simulink model "W04_1_straight"  (R2024b)
settings: Solver=FixedStepDiscrete  StartTime=0.0  StopTime=inf  FixedStep=0.05  RelTol=1e-3
values from neighbouring files (symbols this model uses):
  animate = 1    [W04_setup.m]
libraries: ros2lib x5
settings Model: Creator=admin  LastModifiedBy=admin

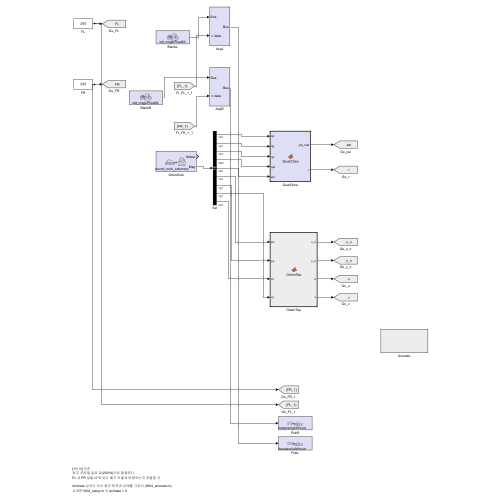
[thumbnail: Simulink's stored preview of the top-level diagram]
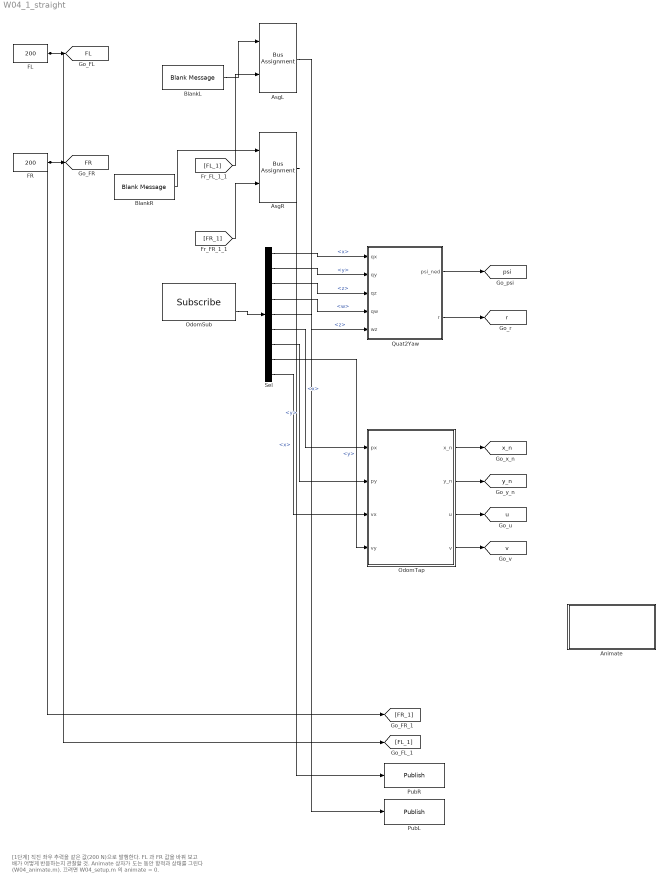
== system W04_1_straight ==
  note: [1단계] 직진
      | 좌우 추력을 같은 값(200 N)으로 발행한다.
      | FL 과 FR 값을 바꿔 보고 배가 어떻게 반응하는지 관찰할 것.
      |
      | Animate 상자가 도는 동안 항적과 상태를 그린다 (W04_animate.m).
      | 끄려면 W04_setup.m 의 animate = 0.
  Animate : Subsystem
  AsgL : BusAssignment  AssignedSignals=data
  AsgR : BusAssignment  AssignedSignals=data
  BlankL : ros2lib/Blank Message  messageClass=Message  entityType=std_msgs/Float64  messageType=std_msgs/Float64  SampleTime=0.05
  BlankR : ros2lib/Blank Message  messageClass=Message  entityType=std_msgs/Float64  messageType=std_msgs/Float64  SampleTime=0.05
  FL : Constant  Value=200
  FR : Constant  Value=200
  OdomSub : ros2lib/Subscribe  topicSource=Specify your own  topic=/wamv/sensors/position/ground_truth_odometry  messageType=nav_msgs/Odometry  sampleTime=0.05  QOSHistory=Keep last  QOSDepth=1  QOSReliability=Reliable  QOSDurability=Volatile  QOSDeadline=Inf  QOSLifespan=Inf  QOSLiveliness=Automatic  QOSLeaseDuration=Inf  QOSAvoidROSNamespaceConventions=off
  OdomTap : MATLAB Function  TreatAsAtomicUnit=on
  PubL : ros2lib/Publish  topicSource=Specify your own  topic=/wamv/thrusters/left/thrust  messageType=std_msgs/Float64  QOSHistory=Keep last  QOSDepth=1  QOSReliability=Reliable  QOSDurability=Volatile  QOSDeadline=Inf  QOSLifespan=Inf  QOSLiveliness=Automatic  QOSLeaseDuration=Inf  QOSAvoidROSNamespaceConventions=off
  PubR : ros2lib/Publish  topicSource=Specify your own  topic=/wamv/thrusters/right/thrust  messageType=std_msgs/Float64  QOSHistory=Keep last  QOSDepth=1  QOSReliability=Reliable  QOSDurability=Volatile  QOSDeadline=Inf  QOSLifespan=Inf  QOSLiveliness=Automatic  QOSLeaseDuration=Inf  QOSAvoidROSNamespaceConventions=off
  Quat2Yaw : MATLAB Function  TreatAsAtomicUnit=on
  Sel : BusSelector  OutputSignals=pose.pose.orientation.x,pose.pose.orientation.y,pose.pose.orientation.z,pose.pose.orientation.w,twist.twist.angular.z,pose.pose.position.x,pose.pose.position.y,twist.twist.linear.y,twist.twist.linear.x
  tag scope: FL=global, FR=global, psi=global, r=global, u=global, v=global, x_n=global, y_n=global
  wires:
  BlankL/1 -> AsgL/1
  BlankR/1 -> AsgR/1
  FL/1 -> [FL], [FL_1]
  FR/1 -> [FR], [FR_1]
  OdomSub/2 -> Sel/1
  Sel/1 -> Quat2Yaw/1(qx)  "<x>"
  Sel/2 -> Quat2Yaw/2(qy)  "<y>"
  Sel/3 -> Quat2Yaw/3(qz)  "<z>"
  Sel/4 -> Quat2Yaw/4(qw)  "<w>"
  Sel/5 -> Quat2Yaw/5(wz)  "<z>"
  Sel/6 -> OdomTap/1(px)  "<x>"
  Sel/7 -> OdomTap/2(py)  "<y>"
  Sel/9 -> OdomTap/3(vx)  "<x>"
  Sel/8 -> OdomTap/4(vy)  "<y>"
  OdomTap/1(x_n) -> [x_n]
  OdomTap/2(y_n) -> [y_n]
  OdomTap/3(u) -> [u]
  OdomTap/4(v) -> [v]
  Quat2Yaw/1(psi_ned) -> [psi]
  Quat2Yaw/2(r) -> [r]
  [FR_1] -> AsgR/2
  [FL_1] -> AsgL/2
  AsgR/1 -> PubR/1
  AsgL/1 -> PubL/1

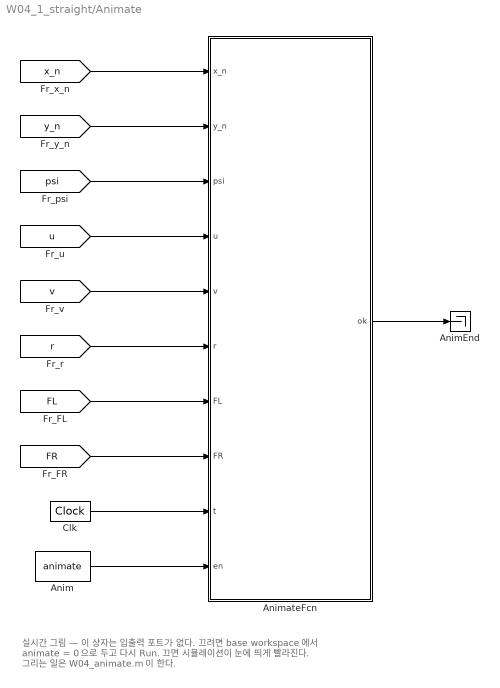
== system W04_1_straight/Animate ==
  note: 실시간 그림 — 이 상자는 입출력 포트가 없다.
      | 끄려면 base workspace 에서  animate = 0  으로 두고 다시 Run.
      | 끄면 시뮬레이션이 눈에 띄게 빨라진다.
      | 그리는 일은 W04_animate.m 이 한다.
  Anim : Constant  Value=animate
  AnimEnd : Terminator
  AnimateFcn : MATLAB Function  TreatAsAtomicUnit=on
  Clk : DigitalClock  SampleTime=0.05
  wires:
  [x_n] -> AnimateFcn/1(x_n)
  [y_n] -> AnimateFcn/2(y_n)
  [psi] -> AnimateFcn/3(psi)
  [u] -> AnimateFcn/4(u)
  [v] -> AnimateFcn/5(v)
  [r] -> AnimateFcn/6(r)
  [FL] -> AnimateFcn/7(FL)
  [FR] -> AnimateFcn/8(FR)
  Clk/1 -> AnimateFcn/9(t)
  Anim/1 -> AnimateFcn/10(en)
  AnimateFcn/1(ok) -> AnimEnd/1

== matlab function W04_1_straight/OdomTap ==
  data: px input; x_n output; py input; vx input; vy input; y_n output; u output; v output
function [x_n, y_n, u, v] = OdomTap(px, py, vx, vy)
%#codegen
% Ground truth odometry -> the numbers the live plot draws.
% Display only: nothing here feeds the controller.
x_n = py;      % ENU y is north
y_n = px;      % ENU x is east
u   =  vx;     % surge is the same in FLU and NED body axes
v   = -vy;     % FLU +y is port, NED +y is starboard

== matlab function W04_1_straight/Quat2Yaw ==
  data: qx input; psi_ned output; qy input; qz input; qw input; wz input; r output
function [psi_ned, r] = Quat2Yaw(qx, qy, qz, qw, wz)
%#codegen
% ROS quaternion (ENU body) -> NED heading [rad] and yaw rate [rad/s]
yaw_enu = atan2(2*(qw*qz + qx*qy), 1 - 2*(qy*qy + qz*qz));
psi = pi/2 - yaw_enu;
psi_ned = atan2(sin(psi), cos(psi));   % wrap to [-pi, pi]

% psi_ned = pi/2 - yaw_enu  ->  d(psi_ned)/dt = -d(yaw_enu)/dt.
% ENU is z-up and NED is z-down, so the turn direction flips.
r = -wz;

== matlab function W04_1_straight/Animate/AnimateFcn ==
  data: x_n input; y_n input; psi input; u input; ok output; v input; r input; FL input; FR input; t input; en input
function ok = AnimateFcn(x_n, y_n, psi, u, v, r, FL, FR, t, en)
%#codegen
% 실시간 그림. MATLAB Function 블록은 그림을 그리지 못하므로 그리는 함수를
% extrinsic 으로 선언한다 — 코드를 만들지 않고 평범한 MATLAB 을 부른다.
% en = base workspace 의 animate (0 이면 그리지 않는다).
coder.extrinsic('W04_animate');
ok = 1;
if en > 0.5
    W04_animate(x_n, y_n, psi, u, v, r, FL, FR, NaN, NaN, t);
end
